simulink model "ControllerObserver"  (R2024a)
settings: Solver=VariableStepAuto  StartTime=0.0  StopTime=10.0  RelTol=1e-3
values from neighbouring files (symbols this model uses):
  Ao = A - L*C    [values.m]
  beta = 3.5    [values.m]
  Bo = [B L]    [values.m]
  Co = eye(size(A))    [values.m]
  Do = zeros(size(A,1),2)    [values.m]
  g = 9.81    [values.m]
  h = H * 0.567    (= 0.9072)    [values.m]
  H = 1.60    (= 1.6)    [values.m]
  Is = m * (K*H).^2    [values.m]
  K = 0.448    [values.m]
  K_ack = -acker(A,B, [-2.5 -3 -10])    [values.m]
  Tmus = 0.1    [values.m]
undefined symbols (not defined in the file or in its folder): ueq, xeq
settings Model: Creator=franc  LastModifiedBy=franc

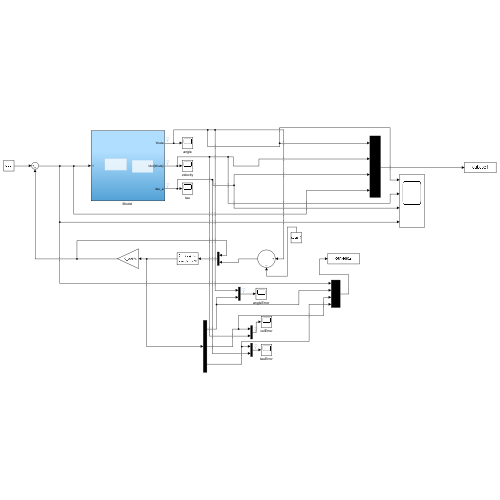
[thumbnail: Simulink's stored preview of the top-level diagram]
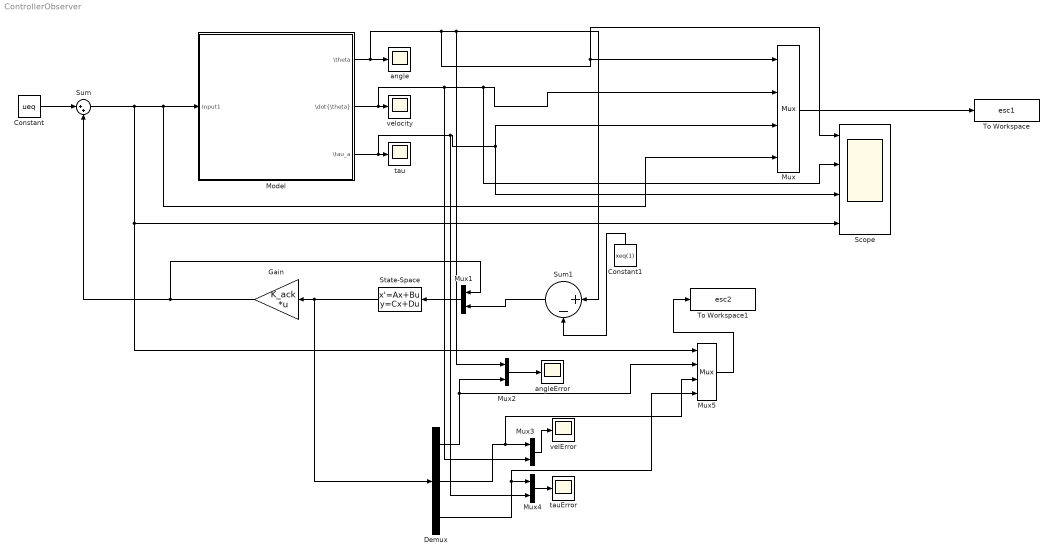
== system ControllerObserver ==
  Constant : Constant  Value=ueq
  Constant1 : Constant  Value=xeq(1)
  Demux : Demux  Outputs=3
  Gain : Gain  Gain=K_ack  Multiplication=Matrix(K*u)
  "Model " : Subsystem
  Mux : Mux
  Mux{1..4} (4 alike) : Mux  Inputs=2
  Mux5 : Mux
  Scope : Scope  NumInputPorts=4
  State-Space : StateSpace  A=Ao  B=Bo  C=Co  D=Do  InitialCondition=[0 0 0]
  Sum : Sum  Inputs=|++
  Sum1 : Sum  Inputs=|+-
  To Workspace : ToWorkspace  VariableName=esc1  SaveFormat=Timeseries  SampleTime=-1
  To Workspace1 : ToWorkspace  VariableName=esc2  SaveFormat=Timeseries  SampleTime=-1
  angle : Scope
  angleError : Scope
  tau : Scope
  tauError : Scope
  velError : Scope
  velocity : Scope
  wires:
  Constant1/1 -> Sum1/2
  Constant/1 -> Sum/1
  Sum/1 -> Mux5/1, Scope/4, Mux/4, "Model "/1(Input1)
  "Model "/2("\\dot{\\theta}") -> Mux3/2, Scope/2, Mux/2, velocity/1
  "Model "/3(\tau_a) -> Mux4/2, Scope/3, Mux/3, tau/1
  Mux/1 -> To Workspace/1
  "Model "/1(\theta) -> Mux2/1, Sum1/1, Scope/1, Mux/1, angle/1
  Gain/1 -> Mux1/1, Sum/2
  State-Space/1 -> Demux/1, Gain/1
  Sum1/1 -> Mux1/2
  Mux1/1 -> State-Space/1
  Demux/1 -> Mux2/2, Mux5/2
  Mux2/1 -> angleError/1
  Mux5/1 -> To Workspace1/1
  Demux/2 -> Mux5/3, Mux3/1
  Demux/3 -> Mux5/4, Mux4/1
  Mux3/1 -> velError/1
  Mux4/1 -> tauError/1

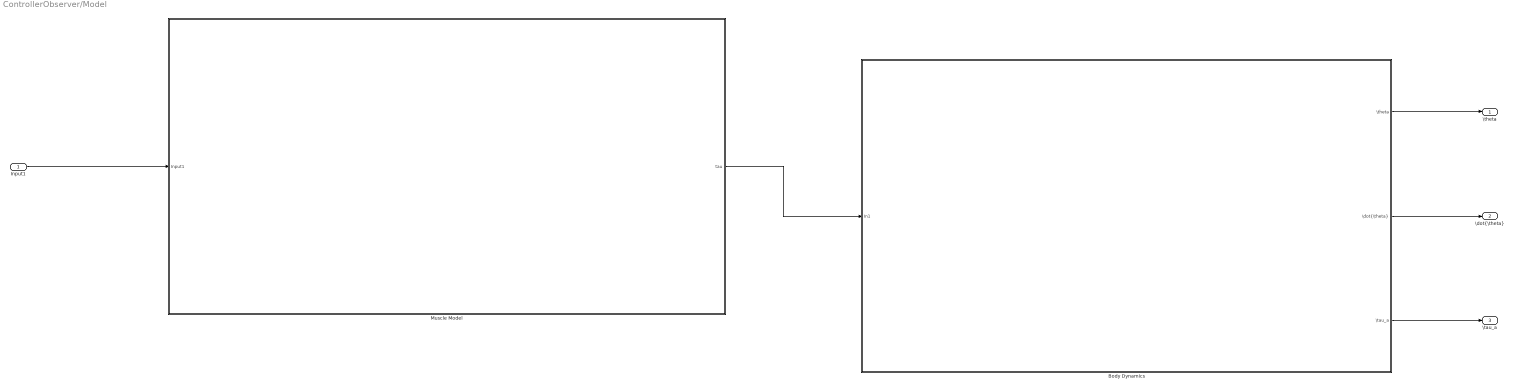
== system ControllerObserver/Model  ==
  Input1 : Inport
  Body Dynamics : Subsystem
      mask Display: image('body2.png');
  Muscle Model : Subsystem
      mask Display: image('muscleModel.png');
  \theta : Outport
  "\\dot{\\theta}" : Outport  Port=2
  \tau_a : Outport  Port=3
  wires:
  Input1/1 -> Muscle Model/1(Input1)
  Body Dynamics/1(\theta) -> \theta/1
  Muscle Model/1(tau) -> Body Dynamics/1(In1)
  Body Dynamics/2("\\dot{\\theta}") -> "\\dot{\\theta}"/1
  Body Dynamics/3(\tau_a) -> \tau_a/1

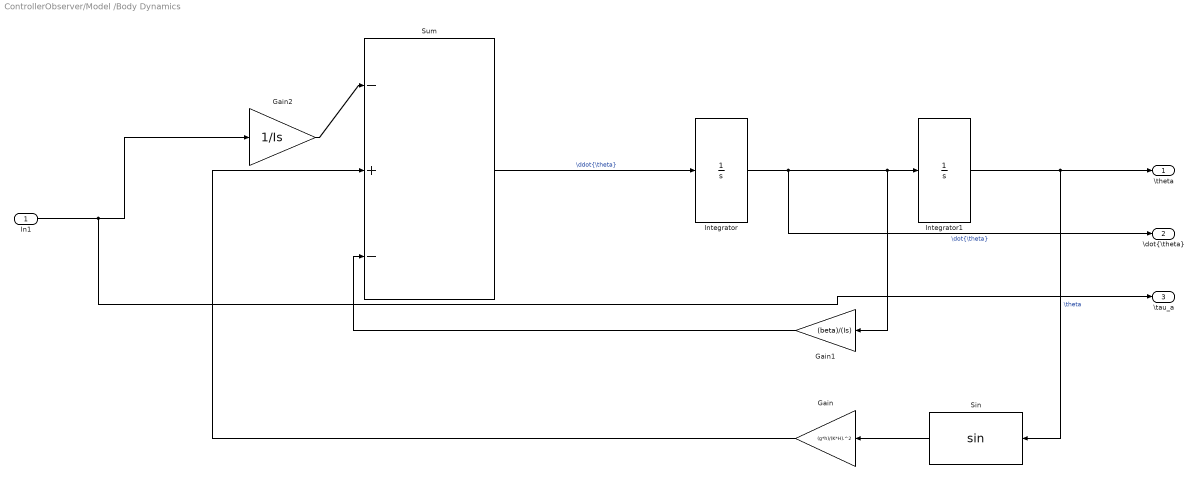
== system ControllerObserver/Model /Body Dynamics ==
  In1 : Inport
  Gain : Gain  Gain=(g*h)/(K*H).^2
  Gain1 : Gain  Gain=(beta)/(Is)
  Gain2 : Gain  Gain=1/Is
  Integrator : Integrator
  Integrator1 : Integrator  InitialCondition=0.1
  Sin : Trigonometry
  Sum : Sum  Inputs=|-+-
  \theta : Outport
  "\\dot{\\theta}" : Outport  Port=2
  \tau_a : Outport  Port=3
  wires:
  Sum/1 -> Integrator/1  "\\ddot{\\theta}"
  Integrator1/1 -> \theta/1, Sin/1  "\\theta"
  Gain1/1 -> Sum/3
  Integrator/1 -> "\\dot{\\theta}"/1, Gain1/1, Integrator1/1  "\\dot{\\theta}"
  Sin/1 -> Gain/1
  Gain2/1 -> Sum/1
  Gain/1 -> Sum/2
  In1/1 -> \tau_a/1, Gain2/1

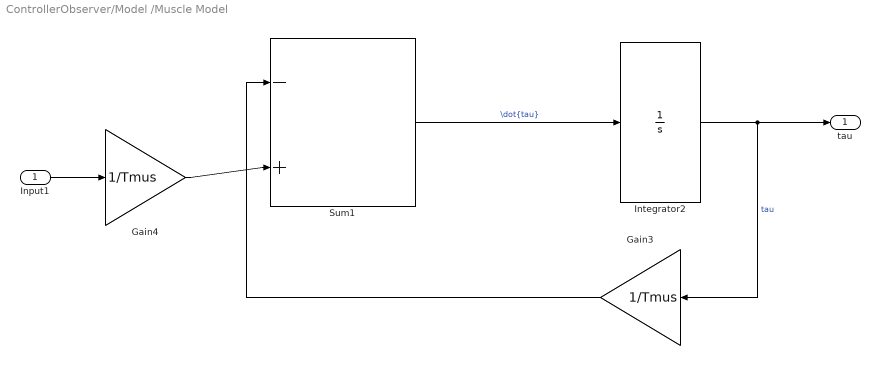
== system ControllerObserver/Model /Muscle Model ==
  Input1 : Inport
  Gain3 : Gain  Gain=1/Tmus
  Gain4 : Gain  Gain=1/Tmus
  Integrator2 : Integrator
  Sum1 : Sum  Inputs=|-+
  tau : Outport
  wires:
  Gain3/1 -> Sum1/1
  Integrator2/1 -> tau/1, Gain3/1  "tau"
  Sum1/1 -> Integrator2/1  "\\dot{tau}"
  Input1/1 -> Gain4/1
  Gain4/1 -> Sum1/2
